simulink model "SPREZYNA_PODWOJNA"  (R2023b)
settings: Solver=VariableStepAuto  StartTime=0.0  StopTime=50  RelTol=1e-3
settings Model: Creator=z1186362  LastModifiedBy=z1186362

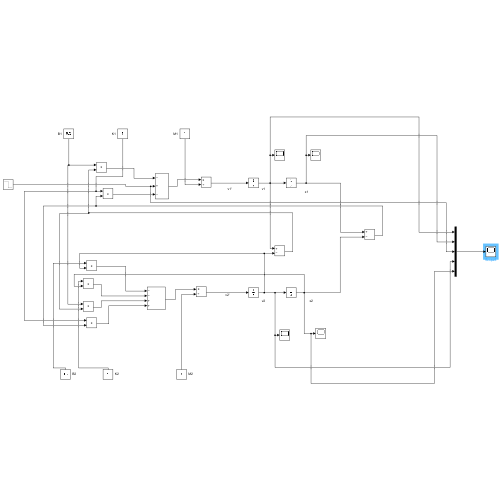
[thumbnail: Simulink's stored preview of the top-level diagram]
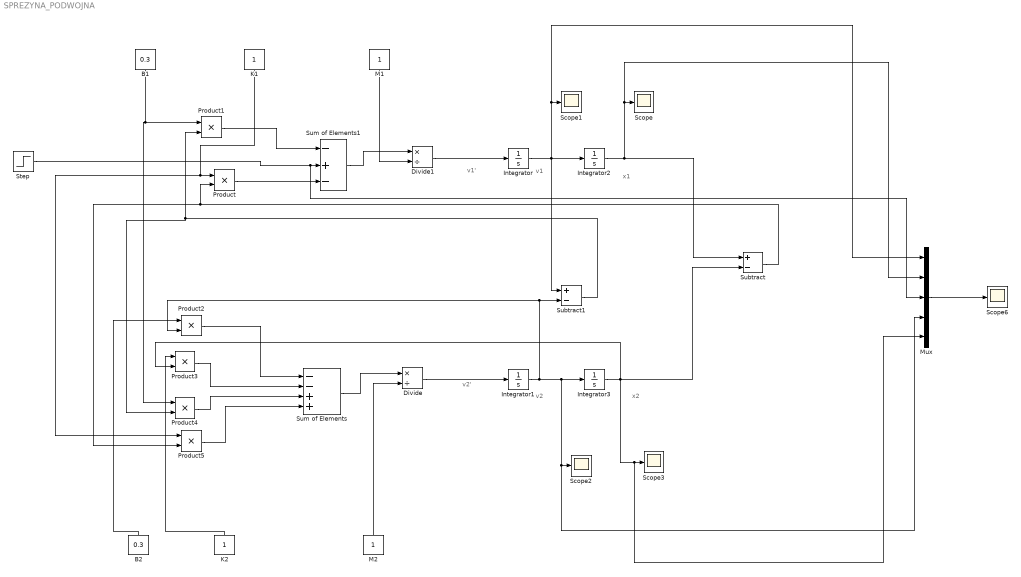
== system SPREZYNA_PODWOJNA ==
  note: v2
  note: v1
  note: v2'
  note: v1'
  note: x1
  note: x2
  B1 : Constant  Value=0.3
  B2 : Constant  Value=0.3
  Divide : Product  Inputs=*/
  Divide1 : Product  Inputs=*/
  Integrator{,1..3} (4 alike) : Integrator
  K1 : Constant
  K2 : Constant
  M1 : Constant
  M2 : Constant
  Mux : Mux  Inputs=5
  Product{,1..5} (6 alike) : Product
  Scope{,1..3,6} (5 alike) : Scope
  Step : Step  Time=10  After=-1  SampleTime=0
  Subtract : Sum  Inputs=+-
  Subtract1 : Sum  Inputs=+-
  Sum of Elements : Sum  Inputs=--++
  Sum of Elements1 : Sum  Inputs=-+-
  wires:
  M2/1 -> Divide/2
  Sum of Elements1/1 -> Divide1/1
  M1/1 -> Divide1/2
  Sum of Elements/1 -> Divide/1
  Divide1/1 -> Integrator/1
  Integrator/1 -> Subtract1/1, Mux/1, Scope1/1, Integrator2/1
  Divide/1 -> Integrator1/1
  Integrator1/1 -> Product2/2, Subtract1/2, Mux/4, Scope2/1, Integrator3/1
  Step/1 -> Mux/3, Sum of Elements1/2
  Product/1 -> Sum of Elements1/3
  Product1/1 -> Sum of Elements1/1
  Product2/1 -> Sum of Elements/1
  Product3/1 -> Sum of Elements/2
  Product4/1 -> Sum of Elements/3
  Product5/1 -> Sum of Elements/4
  B1/1 -> Product4/1, Product1/1
  Integrator2/1 -> Mux/2, Scope/1, Subtract/1
  Integrator3/1 -> Mux/5, Scope3/1, Product3/2, Subtract/2
  Subtract1/1 -> Product4/2, Product1/2
  K1/1 -> Product5/1, Product/1
  Subtract/1 -> Product5/2, Product/2
  B2/1 -> Product2/1
  K2/1 -> Product3/1
  Mux/1 -> Scope6/1
